simulink model "sim_HIL_code_algorithm"  (R2023a)
settings: Solver=FixedStepAuto  StartTime=0.0  StopTime=Inf  FixedStep=0.001  RelTol=1e-3  EnableMultiTasking=on
model workspace (MAT data in the model file):
  Fe = 0.02
  I_max = 0.5
  J = 0.01
  Ke = 0.75
  Kt = 0.75
  L = 1.1
  R = 5.2
  theta_max = 5
  u_max = 12
libraries: arduinolib x4, sldrtlib x1
settings Model: ExtModeTrigDuration=2  Creator=Tu  LastModifiedBy=Tu
settings OptimizationCC: EnhancedBackFolding=on  PassReuseOutputArgsAs=Individual arguments  ZeroExternalMemoryAtStartup=off  ZeroInternalMemoryAtStartup=off  MaxStackSize=64  OptimizeBlockOrder=speed  DifferentSizesBufferReuse=on  OptimizationCustomize=off  EfficientTunableParamExpr=on
settings DebuggingCC: ParameterPrecisionLossMsg=none  ParameterTunabilityLossMsg=error
settings HardwareCC: ProdBitPerInt=16  ProdBitPerPointer=16  ProdBitPerSizeT=16  ProdBitPerPtrDiffT=16  ProdLargestAtomicFloat=None  ProdWordSize=8  ProdHWDeviceType=Atmel->AVR
settings SFSimCC: MATLABDynamicMemAlloc=off
settings RTWCC: Description=Embedded Coder  SystemTargetFile=ert.tlc  HardwareBoard=Arduino Mega 2560  TemplateMakefile=ert_default_tmf  Toolchain=Arduino AVR  BuildConfiguration=Faster Runs
settings CodeAppCC: ForceParamTrailComments=on  IgnoreCustomStorageClasses=off  OperatorAnnotations=on  SimulinkDataObjDesc=on  SFDataObjDesc=on  InsertBlockDesc=on
settings ERTTargetCC: SupportContinuousTime=on  SupportVariableSizeSignals=on  ExtModeTransport=3  ExtModeStaticAlloc=on  ExtModeAutomaticAllocSize=off  ExtModeStaticAllocSize=2048  ExtModeMexFile=ext_xcp  ExtModeIntrfLevel=Level2 - Open

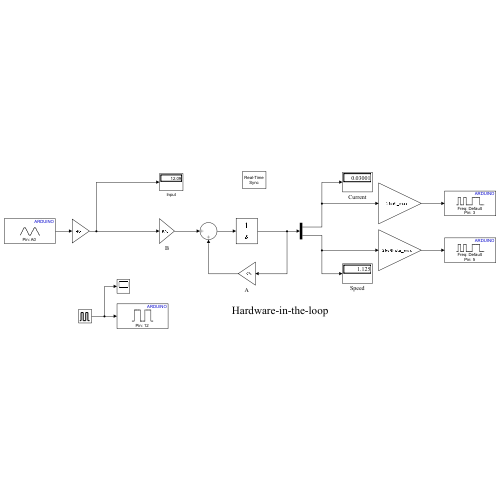
[thumbnail: Simulink's stored preview of the top-level diagram]
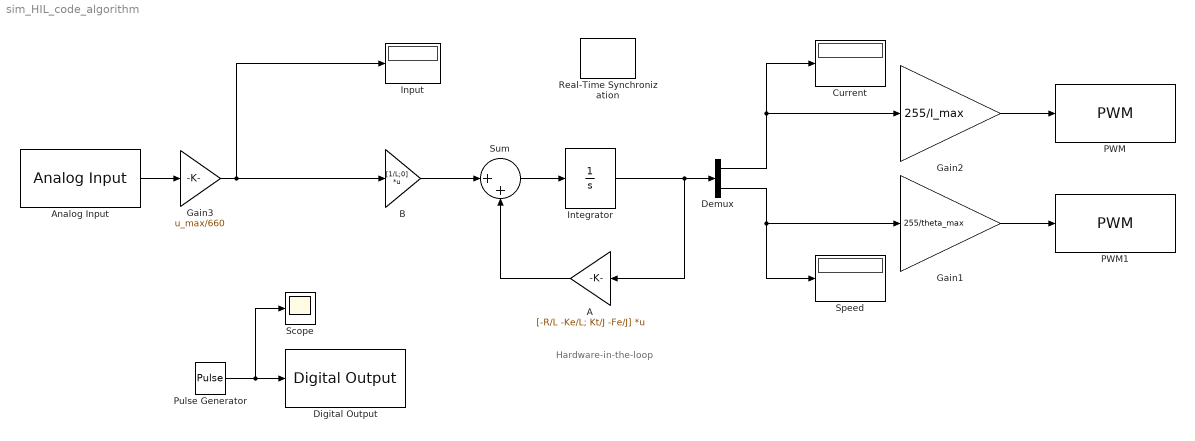
== system sim_HIL_code_algorithm ==
  note: Hardware-in-the-loop
  A : Gain  Gain=[-R/L -Ke/L; Kt/J -Fe/J]  Multiplication=Matrix(K*u)
  Analog Input : arduinolib/Analog Input  pinNumber=0  ReadResultsOnly=off  ConversionTriggerSource=Software  ExternalTriggerType=uint32( 0 )  OutputDataType=uint16  EnableConversionCompleteNotify=off  EnableOuputStatus=off  SampleTime=-1  blockPlatform=arduino
  B : Gain  Gain=[1/L;0]  Multiplication=Matrix(K*u)
  Current : Display
  Demux : Demux  Outputs=2
  Digital Output : arduinolib/Digital Output  pinNumber=12  Direction=output  blockPlatform=arduino
  Gain1 : Gain  Gain=255/theta_max
  Gain2 : Gain  Gain=255/I_max
  Gain3 : Gain  Gain=u_max/660
  Input : Display
  Integrator : Integrator
  PWM : arduinolib/PWM  pinNumber=3  frequencyType=Default  desiredFrequency=490.2  achievableFrequency=490.2
  PWM1 : arduinolib/PWM  pinNumber=5  frequencyType=Default  desiredFrequency=490.2  achievableFrequency=490.2
  Pulse Generator : DiscretePulseGenerator  PulseType=Time based  Period=0.01  PulseWidth=50
  Real-Time Synchronization : sldrtlib/Real-Time Synchronization  SampleTime=0.01  MaxMissedTicks=100000  ShowMissedTicks=off  YieldWhenWaiting=off
  Scope : Scope
  Speed : Display
  Sum : Sum  Inputs=|++
  wires:
  Sum/1 -> Integrator/1
  B/1 -> Sum/1
  A/1 -> Sum/2
  Integrator/1 -> A/1, Demux/1
  Gain2/1 -> PWM/1
  Gain1/1 -> PWM1/1
  Demux/1 -> Current/1, Gain2/1
  Demux/2 -> Gain1/1, Speed/1
  Analog Input/1 -> Gain3/1
  Pulse Generator/1 -> Scope/1, Digital Output/1
  Gain3/1 -> B/1, Input/1
